simulink model "Braccio_trajectory_tracking"  (R2021a)
settings: Solver=FixedStepAuto  StartTime=0.0  StopTime=inf  RelTol=1e-3  EnableMultiTasking=on
InitFcn:
  | cBase=90;
  | cShoulder=90;
  | cElbow=90;
  | cWristVer=90;
  | cWristRot=90;
  | cGripper=73;
values from neighbouring files (symbols this model uses):
  adMotorLimits = [ 0, 180 ... (first row only)    [initSim.m]
  eePos = ppval(traj,x)    [IK_trajectory_tracking.m]
  JointCommands = zeros(size(eePos,2),numJoints)    [IK_trajectory_tracking.m]
  wayPoints = wayPoints'    [IK_trajectory_tracking.m]
libraries: arduinolib x7
settings Model: SILPILModeSetting=veronly  ExtModeTrigDuration=2  Creator=loris  LastModifiedBy=angelo
settings OptimizationCC: EnhancedBackFolding=on  PassReuseOutputArgsAs=Individual arguments  ZeroExternalMemoryAtStartup=off  ZeroInternalMemoryAtStartup=off  MaxStackSize=64  OptimizeBlockOrder=speed  DifferentSizesBufferReuse=on  OptimizationCustomize=off  EfficientTunableParamExpr=on
settings DebuggingCC: ParameterTunabilityLossMsg=error
settings HardwareCC: ProdBitPerInt=16  ProdBitPerPointer=16  ProdBitPerSizeT=16  ProdBitPerPtrDiffT=16  ProdLargestAtomicFloat=None  ProdWordSize=8  ProdHWDeviceType=Atmel->AVR
settings SFSimCC: MATLABDynamicMemAlloc=off
settings RTWCC: SystemTargetFile=ert.tlc  HardwareBoard=Arduino Mega 2560  TemplateMakefile=ert_default_tmf  Toolchain=Arduino AVR  BuildConfiguration=Faster Runs
settings CodeAppCC: ForceParamTrailComments=on  IgnoreCustomStorageClasses=off  OperatorAnnotations=on  SimulinkDataObjDesc=on  SFDataObjDesc=on  InsertBlockDesc=on
settings ERTTargetCC: SupportContinuousTime=on  SupportVariableSizeSignals=on  ExtModeStaticAllocSize=2048

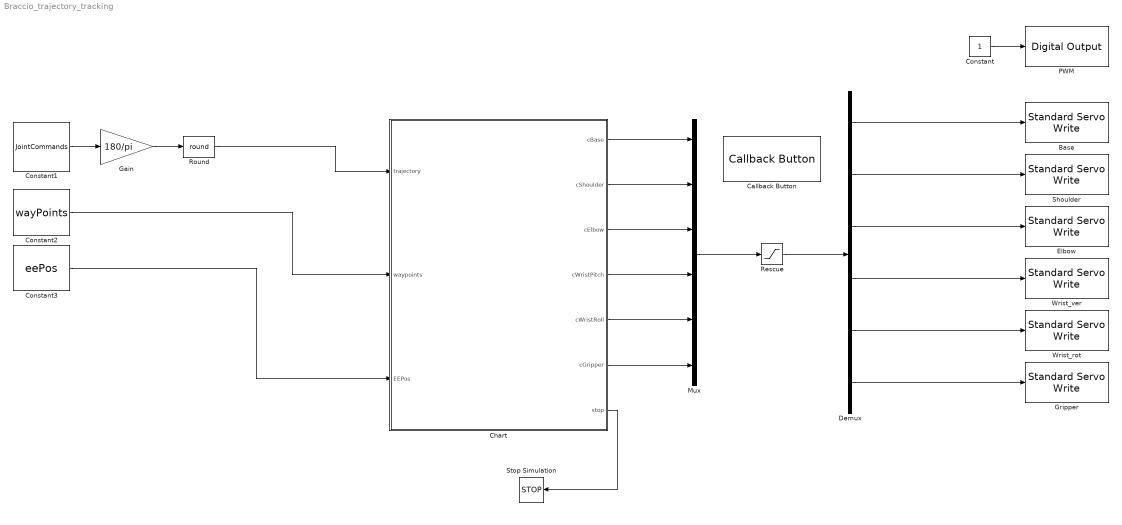
== system Braccio_trajectory_tracking ==
  Base : arduinolib/Standard Servo Write  pinNumber=11  ServoIndex=0  blockPlatform=ARDUINO
  Callback Button : CallbackButton  ButtonText=Load MotorLimits
      settings: ClickFcn=|
      | adMotorLimits = [ 0, 180;
      |                  15, 165;
      |                   0, 180;
      |                   0, 180;
      |                   0, 180;
      |                  10,  73;
      | ];
  Chart : Stateflow chart  TreatAsAtomicUnit=on
  Constant : Constant
  Constant1 : Constant  Value=JointCommands
  Constant2 : Constant  Value=wayPoints
  Constant3 : Constant  Value=eePos
  Demux : Demux  Outputs=6
  Elbow : arduinolib/Standard Servo Write  pinNumber=9  ServoIndex=1  blockPlatform=ARDUINO
  Gain : Gain  Gain=180/pi
  Gripper : arduinolib/Standard Servo Write  pinNumber=3  ServoIndex=2  blockPlatform=ARDUINO
  Mux : Mux  Inputs=6
  PWM : arduinolib/Digital Output  pinNumber=12  Direction=output  blockPlatform=arduino
  Rescue : Saturate  UpperLimit=adMotorLimits(:,2)  LowerLimit=adMotorLimits(:,1)
  Round : Rounding  Operator=round
  Shoulder : arduinolib/Standard Servo Write  pinNumber=10  ServoIndex=3  blockPlatform=ARDUINO
  Stop Simulation : Stop
  Wrist_rot : arduinolib/Standard Servo Write  pinNumber=5  ServoIndex=4  blockPlatform=ARDUINO
  Wrist_ver : arduinolib/Standard Servo Write  pinNumber=6  ServoIndex=5  blockPlatform=ARDUINO
  wires:
  Constant/1 -> PWM/1
  Constant1/1 -> Gain/1
  Gain/1 -> Round/1
  Constant2/1 -> Chart/2(waypoints)
  Round/1 -> Chart/1(trajectory)
  Constant3/1 -> Chart/3(EEPos)
  Chart/7(stop) -> Stop Simulation/1
  Demux/1 -> Base/1
  Demux/2 -> Shoulder/1
  Demux/3 -> Elbow/1
  Demux/4 -> Wrist_ver/1
  Demux/5 -> Wrist_rot/1
  Demux/6 -> Gripper/1
  Mux/1 -> Rescue/1
  Rescue/1 -> Demux/1
  Chart/6(cGripper) -> Mux/6
  Chart/5(cWristRoll) -> Mux/5
  Chart/4(cWristPitch) -> Mux/4
  Chart/3(cElbow) -> Mux/3
  Chart/2(cShoulder) -> Mux/2
  Chart/1(cBase) -> Mux/1

== stateflow chart Braccio_trajectory_tracking/Chart ==
  settings: executeAtInitialization=1
  state SetConfiguration
    entry:
    counter=0;
    cBase=trajectory(currentState,1);
    cShoulder=trajectory(currentState,2);
    cElbow=trajectory(currentState,3);
    cWristPitch=trajectory(currentState,4);
    during:
    counter=temporalCount(msec);
  state Inizialization
    entry:
    cBase=90;
    cShoulder=90;
    cElbow=90;
    cWristPitch=90;
    cWristRoll=90;
    cGripper=10;
    endMotion=0;
    stop=0;
    counter=0;
    GripperCommand=0;
    currentState=1;
    during:
    counter=temporalCount(sec);
  state OpenGripper
    entry:
    counter=0;
    cGripper=10;
    GripperCommand=0;
    during:
    counter=temporalCount(sec);
  state EndMotion
    entry:
    cBase=90
    cShoulder=90;
    cElbow=90;
    cWristPitch=90;
    cWristRoll=0;
    cGripper=73;
    counter=0;
    during:
    counter=temporalCount(sec);
  state ToNextPoint
    entry:
    if currentState<size(trajectory,1)
    currentState=currentState+1;
    endMotion=0;
    else
    endMotion=1;
    end
  state WayPointReached
    entry:
    if GripperCommand==2
    GripperAction=1;
    elseif GripperCommand==1
    GripperAction=0;
    end
  state CloseGripper
    entry:
    counter=0;
    cGripper=73;
    GripperCommand=0;
    during:
    counter=temporalCount(sec);
  state CheckWayPointReached
    entry:
    if abs(EEPos(:,currentState)-waypoints(:,2))<0.01
    GripperCommand=1;
    elseif abs(EEPos(:,currentState)-waypoints(:,4))<0.01
    GripperCommand=2
    end
  state STOP
    entry:
    stop=1;
  (default) -> Inizialization
  CloseGripper -> SetConfiguration : [counter==2]
  Inizialization -> SetConfiguration : [counter==2]
  OpenGripper -> SetConfiguration : [counter==2]
  CheckWayPointReached -> SetConfiguration [order 1] : [GripperCommand==0]
  SetConfiguration -> ToNextPoint : [counter==50]
  WayPointReached -> OpenGripper [order 1] : [GripperAction==1]
  ToNextPoint -> EndMotion [order 2] : [endMotion==1]
  CheckWayPointReached -> WayPointReached [order 2] : [GripperCommand~=0]
  WayPointReached -> CloseGripper [order 2] : [GripperAction==0]
  ToNextPoint -> CheckWayPointReached [order 1] : [endMotion==0]
  EndMotion -> STOP : [counter==2]
  data: trajectory input; waypoints input; cBase output; cShoulder output; cElbow output; cWristPitch output; cWristRoll output; cGripper output; counter local; currentState local; EEPos input; GripperCommand local; GripperAction local; stop output; endMotion local
